simulink model "PROB_9_BLDC_MOTOR"  (R2020b)
settings: Solver=VariableStepAuto  StartTime=0.0  StopTime=10.0  RelTol=1e-3
model workspace (MAT data in the model file):
  den = [0.0001 0.014]
  den1 = [0.0002 0.004586]
  kT = 0.0275
  ke = 0.0275
  num = 1
  num1 = 1
settings Model: Creator=intel  LastModifiedBy=intel

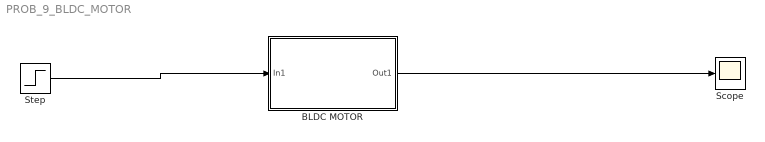
== system PROB_9_BLDC_MOTOR ==
  BLDC MOTOR : Subsystem  TreatAsAtomicUnit=on
      mask Display: image('bldc_motor.png'); % Use "Edit Image" on toolstrip to change.
  Scope : Scope
  Step : Step  SampleTime=0
  wires:
  Step/1 -> BLDC MOTOR/1(In1)
  BLDC MOTOR/1(Out1) -> Scope/1

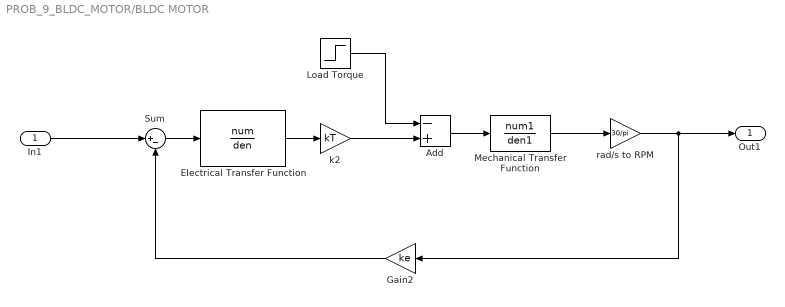
== system PROB_9_BLDC_MOTOR/BLDC MOTOR ==
  In1 : Inport
  " Mechanical Transfer Function" : TransferFcn  Numerator=num1  Denominator=den1
  Add : Sum  Inputs=-+
  Electrical Transfer Function : TransferFcn  Numerator=num  Denominator=den
  Gain2 : Gain  Gain=ke
  Load Torque : Step  SampleTime=0
  Sum : Sum  Inputs=|+-
  "k2 " : Gain  Gain=kT
  rad/s to RPM : Gain  Gain=30/pi
  Out1 : Outport
  wires:
  In1/1 -> Sum/1
  Electrical Transfer Function/1 -> "k2 "/1
  Sum/1 -> Electrical Transfer Function/1
  Add/1 -> " Mechanical Transfer Function"/1
  Gain2/1 -> Sum/2
  " Mechanical Transfer Function"/1 -> rad/s to RPM/1
  rad/s to RPM/1 -> Out1/1, Gain2/1
  Load Torque/1 -> Add/1
  "k2 "/1 -> Add/2
